simulink model "sf_seqrec"  (R2017b)
settings: Solver=FixedStepDiscrete  StartTime=0.0  StopTime=10.0  RelTol=1e-3  EnableMultiTasking=on
undefined symbols (not defined in the file): sigbuilder_block
Description:
  | This demo shows how Mealy and Moore machines can be used in signal processing applications; in this case, for sequence recognition.  In the Moore machine, actions can only be state actions, whereas in the Mealy machine, actions can only be condition actions.
  | 
  | The two Stateflow(R) charts are used to find the sequence 1,2,1,3 in the input signal from Signal Builder.  The status of the sequence recognition is logged in the output variable "state."  If the sequence is found, the variable seqFound is set to 1.  On running the simulation and opening the scopes, notice that the Moore output is delayed by one time step.  This is because the output from a Moore machine is based on the state from the previous time step, and the output from a Mealy machine is based on the state from the previous time step and the current input.
  | 
  | Ref: Digital Design: From Gates to Intelligent Machines, 2006 by Bruce F. Katz
settings Model: Creator=The MathWorks, Inc.  LastModifiedBy=The MathWorks, Inc.
settings DataIOCC: LimitDataPoints=on  SaveFormat=Array
settings OptimizationCC: ExpressionDepthLimit=2147483647  InitFltsAndDblsToZero=on  EfficientMapNaN2IntZero=off  LifeSpan=1
settings DebuggingCC: SaveWithParameterizedLinksMsg=none  UnderspecifiedInitializationDetection=Classic  MergeDetectMultiDrivingBlocksExec=none  SignalResolutionControl=TryResolveAllWithWarning  SolverPrmCheckMsg=warning  FcnCallInpInsideContextMsg=warning  AllowSymbolicDim=off  StateNameClashWarn=warning  StrictBusMsg=Warning  SFUnexpectedBacktrackingDiag=warning  SFNoUnconditionalDefaultTransitionDiag=warning  SFExecutionAtInitializationDiag=none
settings HardwareCC: ProdBitPerPointer=32  ProdBitPerSizeT=32  ProdBitPerPtrDiffT=32  ProdLargestAtomicFloat=None  ProdIntDivRoundTo=Undefined  ProdEndianess=Unspecified  ProdWordSize=32  ProdHWDeviceType=32-bit Generic
settings ModelReferenceCC: PropagateSignalLabelsOutOfModel=off
settings SFSimCC: SimParseCustomCode=off  MATLABDynamicMemAlloc=off
settings RTWCC: SystemTargetFile=ert.tlc  GenCodeOnly=on  TemplateMakefile=ert_default_tmf  Description=Real-Time Workshop Embedded Coder (no auto configuration)
settings CodeAppCC: IgnoreCustomStorageClasses=off  CustomSymbolStrGlobalVar=$N$M  CustomSymbolStrType=$N$M  CustomSymbolStrFcn=$N$M$F  CustomSymbolStrMacro=$N$M  StateflowObjectComments=on  InternalIdentifier=Classic
settings ERTTargetCC: TargetFcnLib=ansi_tfl_tmw.mat  MultiwordLength=2048  GenerateSampleERTMain=on  IncludeMdlTerminateFcn=off  SupportContinuousTime=on  ERTCustomFileTemplate=example_file_process.tlc  ConvertIfToSwitch=off  SuppressUnreachableDefaultCases=off
settings ConfigComp: CovMetricSettings=dw  CovHtmlReporting=on  CovSaveCumulativeToWorkspaceVar=on  CovSaveSingleToWorkspaceVar=on  CovExternalEMLEnable=off  CovSFcnEnable=off

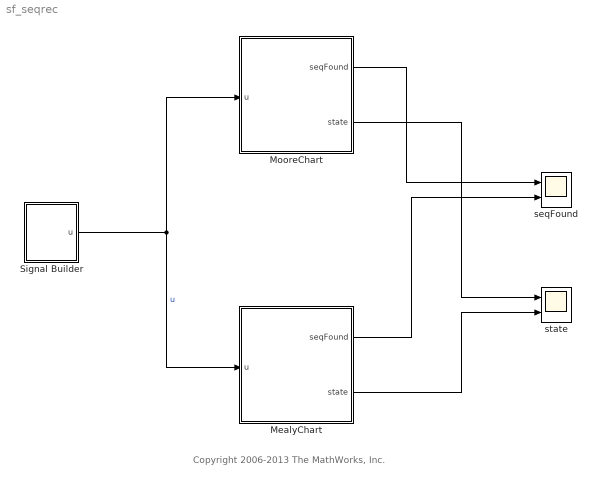
== system sf_seqrec ==
  note: Copyright 2006-2013 The MathWorks, Inc.
  MealyChart : Stateflow chart  TreatAsAtomicUnit=on
  MooreChart : Stateflow chart  TreatAsAtomicUnit=on
  Signal Builder : Subsystem  Tag=STV Subsys  LoadFcn=sigbuilder_block('load');  StartFcn=sigbuilder_block('start');  StopFcn=sigbuilder_block('stop');  ClipboardFcn=sigbuilder_block('clipboard');  mask(Sigbuilder block){tuvar=[0:10]}
      mask help: Sigbuilder GUI
      mask init:
      | if ~strcmp(get_param(bdroot(gcbh),'SimulationStatus'),'stopped') tuvar = sigbuilder_block('maskInit'); end
      settings: CopyFcn=sigbuilder_block('copy');  DeleteFcn=sigbuilder_block('delete');  ModelCloseFcn=sigbuilder_block('modelClose');  PreSaveFcn=sigbuilder_block('preSave');  PauseFcn=sigbuilder_block('pause')  ContinueFcn=sigbuilder_block('continue')  NameChangeFcn=sigbuilder_block('namechange');  OpenFcn=sigbuilder_block('open',[127.5 390 550.5 399.75 ]);  CloseFcn=sigbuilder_block('close');
      mask Display: plot(0, 0, 100, 100,[2, 2, 32, 32, 2], [68, 8, 8, 68, 68],[32, 2], [38, 38], [32, 19, 2],[53, 60, 44], [32, 17, 17, 2],[16, 16, 31, 31]);txt = getActiveGroup(gcbh);text(2, 100, txt,'verticalAlignment', 'top');
  seqFound : Scope  NumInputPorts=2
  state : Scope  NumInputPorts=2
  wires:
  Signal Builder/1(u) -> MooreChart/1(u), MealyChart/1(u)  "u"
  MooreChart/1(seqFound) -> seqFound/1
  MealyChart/1(seqFound) -> seqFound/2
  MealyChart/2(state) -> state/2
  MooreChart/2(state) -> state/1

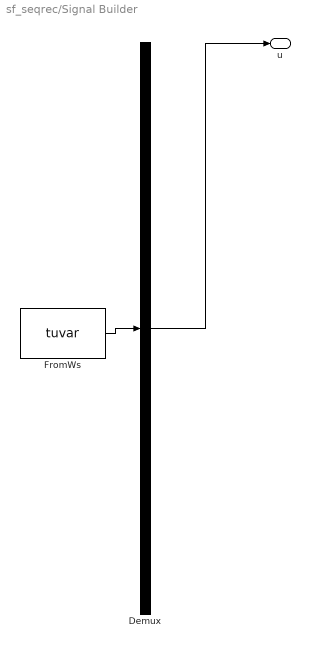
== system sf_seqrec/Signal Builder ==
  Demux : Demux  Tag=STV Demux  Outputs=1
  FromWs : FromWorkspace  Tag=STV FromWs  VariableName=tuvar  SampleTime=0
      SigBuilderData=|
      | common.afterFinalStr = 'Extrapolate'
      | common.sampleTime = 0
      | dataSet.timeRange = [0 10]
      | dataSet.name = 'Group 1'
      | sbobj.Groups.Name = 'Group 1'
      | sbobj.Groups.Signals.Name = 'u'
      | sbobj.Groups.Signals.XData = [0 0.5 1 1.5 2 2 2.5 3 3 3.5 3.5 4 4 4.5 4.5 5 5 5.5 5.5 6 6 6.5 7 7.5 7.5 8 8 8.5 8.5 9 9 9.5 10]
      | sbobj.Groups.Signals.YData = [1 1 1 1 1 0 0 0 1 1 2 2 1 1 3 3 1 1 2 2 1 1 1 1 2 2 1 1 3 3 1 1 1]
  u : Outport  Tag=STV Outport
  wires:
  Demux/1 -> u/1
  FromWs/1 -> Demux/1

== stateflow chart sf_seqrec/MooreChart ==
  settings: updateMethod=DISCRETE  sampleTime=0.5  stateMachineType=MOORE_MACHINE  executeAtInitialization=1  initializeOutput=1
  state s1213
    state=4;
    seqFound=true;
  state s121
    state=3;
  state s12
    state=2;
  state s1
    state=1;
    seqFound=false;
  state s0
    state=0;
    seqFound=false;
  s1213 -> s1 [order 1] : [u==1]
  s121 -> s1 [order 1] : [u==1]
  (default) -> s0
  s1 -> s0 [order 2] : [u~=1]
  s121 -> s12 [order 3] : [u==2]
  s0 -> s1 : [u==1]
  s1 -> s12 [order 1] : [u==2]
  s12 -> s121 [order 1] : [u==1]
  s121 -> s1213 [order 2] : [u==3]
  s1213 -> s0 [order 2]
  s121 -> s0 [order 4]
  s12 -> s0 [order 2]
  data: u input; seqFound output boolean; state output double

== stateflow chart sf_seqrec/MealyChart ==
  settings: updateMethod=DISCRETE  sampleTime=0.5  stateMachineType=MEALY_MACHINE  executeAtInitialization=1  initializeOutput=1
  state s121
  state s1213
  state s0
  state s1
  state s12
  s1213 -> s1 [order 1] : [u==1]...
      | {state=1;...
      | seqFound=false;}
  s121 -> s1 [order 1] : [u==1]...
      | {state=1;}
  (default) -> s0
  s121 -> s12 [order 3] : [u==2]...
      | {state=2;}
  s1 -> s0 [order 2] : [u~=1]{state=0;}
  s12 -> s121 [order 1] : [u==1]...
      | {state=3;}
  s1 -> s12 [order 1] : [u==2]...
      | {state=2;}
  s121 -> s1213 [order 2] : [u==3]...
      | {state=4;...
      | seqFound=true;}
  s0 -> s1 : [u==1]...
      | {state=1;}
  s121 -> s0 [order 4] : {state=0;}
  s12 -> s0 [order 2] : {state=0;}
  s1213 -> s0 [order 2] : {state=0;...
      | seqFound=false;}
  data: u input; seqFound output boolean; state output double
